simulink model "problema3"  (R2021a)
settings: Solver=VariableStepAuto  StartTime=0.0  StopTime=10.0  RelTol=1e-3
values from neighbouring files (symbols this model uses):
  ue = tau_b    [Problema2.m]
  xe = [x1e; x2e; x3e; x4e]    [Problema2.m]
  ye = x1e    (= 0.785398163397)    [Problema2.m]
libraries: cstblocks x1
settings Model: Creator=Santiago  LastModifiedBy=Santiago

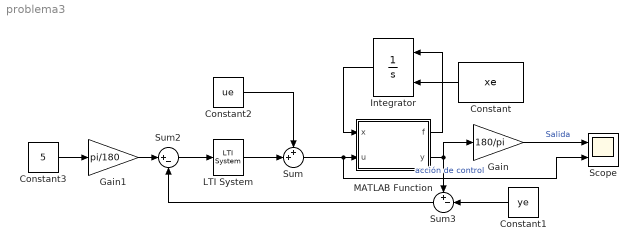
== system problema3 ==
  Constant : Constant  Value=xe
  Constant1 : Constant  Value=ye
  Constant2 : Constant  Value=ue
  Constant3 : Constant  Value=5
  Gain : Gain  Gain=180/pi
  Gain1 : Gain  Gain=pi/180
  Integrator : Integrator  InitialConditionSource=external
  LTI System : cstblocks/LTI System  sys=C  IC=[]
  MATLAB Function : MATLAB Function  TreatAsAtomicUnit=on
  Scope : Scope  NumInputPorts=2
  Sum : Sum  Inputs=++|
  Sum2 : Sum  Inputs=|+-
  Sum3 : Sum  Inputs=+-|
  wires:
  Sum/1 -> Scope/2, MATLAB Function/2(u)  "acción de control"
  Sum2/1 -> LTI System/1
  Constant1/1 -> Sum3/2
  Integrator/1 -> MATLAB Function/1(x)
  Sum3/1 -> Sum2/2
  MATLAB Function/2(y) -> Sum3/1, Gain/1
  LTI System/1 -> Sum/2
  MATLAB Function/1(f) -> Integrator/1
  Constant2/1 -> Sum/1
  Constant/1 -> Integrator/2
  Gain/1 -> Scope/1  "Salida"
  Gain1/1 -> Sum2/1
  Constant3/1 -> Gain1/1

== matlab function problema3/MATLAB Function ==
  data: x input; f output; u input; y output
function [f,y] = fcn(x, u)

f1 = x(2);
f2 = -0.9549 * x(1) + sin(x(1)) - x(2) + x(3);
f3 = x(4);
f4 = -100^2 * x(3) - 2*1*100 *x(4) + 100^2 * u;

f = [f1; f2; f3; f4];

y = x(1);
